simulink model "azfuz_pid"  (Simulink 7.7)
settings: Solver=ode3  StartTime=0.0  StopTime=50  FixedStep=0.1  RelTol=1e-6
PreLoadFcn:
  | load tras_char
values from neighbouring files (symbols this model uses):
  control_a = [-1,-0.975000000000000,-0.950000000000000,-0.925000000000000,-0.900000000000000,-0.875000000000000,-0.850000000000000,-0.825000000000000,-0.800000000000000,-0.775000000000000,-0.750000000000000,-0.725000000000000,-0.700000000000000,-0.675000000000000,-0.650000000000000,-0.625000000000000,-0.600000000000000,-0.575000000000000,-0.550000000000000,-0.525000000000000,-0.500000000000000,-0.4750000000000 ...(+1058 chars)    [main.m]
  force_a = [-1.11662323915155,-1.09378407342940,-1.07265330175950,-1.04325193963191,-1.01132720072323,-0.977223749190414,-0.938313974120250,-0.915271484375000,-0.878089162348878,-0.843089432210708,-0.808883264518567,-0.764209831066494,-0.722158864286485,-0.679419665506261,-0.643924317249568,-0.610622608349525,-0.566994046173359,-0.526776706201425,-0.495851299384715,-0.457681114394430,-0.413805712974957,-0.38 ...(+1125 chars)    [main.m]
  GCE = GE*(Kp-sqrt(Kp^2-4*Ki*Kd))/2/Ki    [main.m]
  GCU = Ki/GE    (= 0.001)    [main.m]
  GE = 1    [main.m]
  GU = Kd/GCE    [main.m]
  rpm_a = [-7339.45782001209,-7212.46690016528,-7085.45931302586,-6928.76328688402,-6788.57281024633,-6657.59465144230,-6511.41380896936,-6365.92031625604,-6207.93597881609,-6041.64663461541,-5911.49080716649,-5761.94058931792,-5622.99053485574,-5477.24984975964,-5308.98813100961,-5148.14194899341,-4993.59811636119,-4838.25096717246,-4657.71766075724,-4490.92806302583,-4332.56953312800,-4153.59004094051,-39 ...(+1020 chars)    [main.m]
  Ts = 0.1    [main.m]
undefined symbols (not defined in the file or in its folder): DiscIntNeverNeededParam
libraries: simulink x2, fuzblock x1
settings Model: Creator=melanholly  LastModifiedBy=melanholly
settings DataIOCC: SignalLoggingName=sigsOut
settings DebuggingCC: SaveWithParameterizedLinksMsg=none  SignalResolutionControl=TryResolveAllWithWarning  SolverPrmCheckMsg=none  MultiTaskDSMMsg=warning  MultiTaskCondExecSysMsg=none  StrictBusMsg=None
settings HardwareCC: TargetUnknown=on
settings RTWCC: IncludeERTFirstTime=on

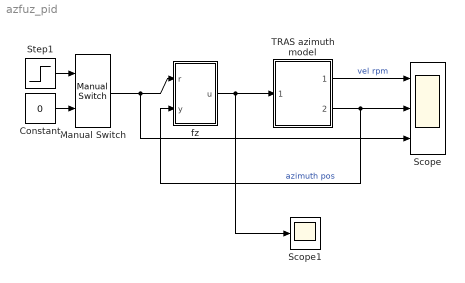
== system azfuz_pid ==
  Constant : Constant  Value=0
  Manual Switch : simulink/Signal Routing/Manual Switch  SystemSampleTime=-1  sw=1  action=0  varsize=off
  Scope : Scope  NumInputPorts=3
      settings: YMin=-5~-5~-5  YMax=5~5~5
  Scope1 : Scope
      settings: TimeRange=12  YMin=0  YMax=1.223758865248227
  Step1 : Step  After=0.3  SampleTime=0
  TRAS azimuth model : Subsystem
  fz : Subsystem
  wires:
  TRAS azimuth model/1(rpm_a) -> Scope/1  "vel rpm"
  TRAS azimuth model/2(pos_am) -> Scope/2, fz/2(y)  "azimuth pos"
  Manual Switch/1 -> Scope/3, fz/1(r)
  Step1/1 -> Manual Switch/1
  Constant/1 -> Manual Switch/2
  fz/1(u) -> TRAS azimuth model/1("ctrl_a "), Scope1/1

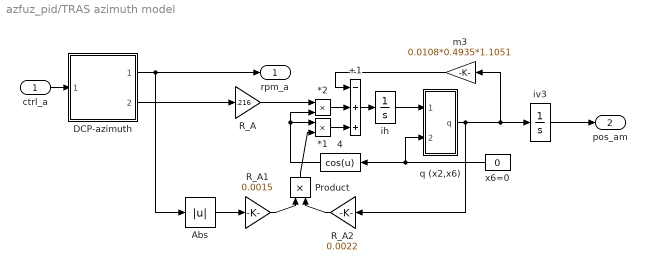
== system azfuz_pid/TRAS azimuth model ==
  "ctrl_a " : Inport
  *1 : Product  SaturateOnIntegerOverflow=on  InputSameDT=on  OutDataTypeStr=Inherit: Same as first input
  *2 : Product  SaturateOnIntegerOverflow=on  InputSameDT=on  OutDataTypeStr=Inherit: Same as first input
  +1 : Sum  Inputs=-++  SaturateOnIntegerOverflow=on  InputSameDT=on  OutDataTypeStr=Inherit: Same as first input
  4 : Fcn  Expr=cos(u)
  Abs : Abs  SaturateOnIntegerOverflow=on
  DCP-azimuth : Subsystem
  Product : Product  SaturateOnIntegerOverflow=on  InputSameDT=on  OutDataTypeStr=Inherit: Same as first input
  R_A : Gain  Gain=.216  OutDataTypeStr=Inherit: Same as input  ParamDataTypeStr=Inherit: Same as input
  R_A1 : Gain  Gain=0.0015  OutDataTypeStr=Inherit: Same as input  ParamDataTypeStr=Inherit: Same as input
  R_A2 : Gain  Gain=0.0022  OutDataTypeStr=Inherit: Same as input  ParamDataTypeStr=Inherit: Same as input
  ih : Integrator
  iv3 : Integrator
  m3 : Gain  Gain=0.0108*0.4935*1.1051  OutDataTypeStr=Inherit: Same as input  ParamDataTypeStr=Inherit: Same as input
  q (x2,x6) : Subsystem
  x6=0 : Constant  Value=0
  rpm_a : Outport
  pos_am : Outport  Port=2
  wires:
  DCP-azimuth/2(FORCE_A) -> R_A/1
  *1/1 -> +1/3
  m3/1 -> +1/1
  4/1 -> *1/1, *2/2
  *2/1 -> +1/2
  ih/1 -> q (x2,x6)/1(x2)
  q (x2,x6)/1(q) -> iv3/1, m3/1, R_A2/1
  R_A/1 -> *2/1
  +1/1 -> ih/1
  x6=0/1 -> q (x2,x6)/2(x6), 4/1
  "ctrl_a "/1 -> DCP-azimuth/1(CTR_A)
  iv3/1 -> pos_am/1
  DCP-azimuth/1(RPM_A) -> rpm_a/1, Abs/1
  Product/1 -> *1/2
  R_A2/1 -> Product/2
  R_A1/1 -> Product/1
  Abs/1 -> R_A1/1

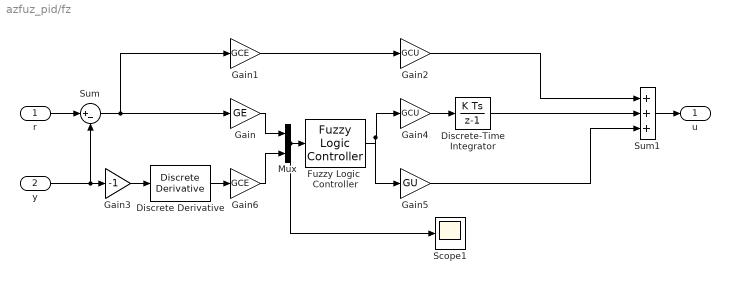
== system azfuz_pid/fz ==
  r : Inport
  y : Inport  Port=2
  Discrete Derivative : simulink/Discrete/Discrete Derivative  SystemSampleTime=-1  gainval=1.0  ICPrevScaledInput=0.0  OutMin=[]  OutMax=[]  OutDataType=fixdt(1, 16)  OutScaling=2^-10  DoSatur=off
  Discrete-Time Integrator : DiscreteIntegrator  SampleTime=Ts  ICPrevOutput=DiscIntNeverNeededParam  ICPrevScaledInput=DiscIntNeverNeededParam
  Fuzzy Logic  Controller : fuzblock/Fuzzy Logic  Controller  SystemSampleTime=-1  fis=FIS
  Gain : Gain  Gain=GE  SampleTime=Ts
  Gain1 : Gain  Gain=GCE  SampleTime=Ts
  Gain2 : Gain  Gain=GCU  SampleTime=Ts
  Gain3 : Gain  Gain=-1  SampleTime=Ts
  Gain4 : Gain  Gain=GCU  SampleTime=Ts
  Gain5 : Gain  Gain=GU  SampleTime=Ts
  Gain6 : Gain  Gain=GCE  SampleTime=Ts
  Mux : Mux  Inputs=2
  Scope1 : Scope
      settings: TimeRange=12  YMin=0  YMax=1.223758865248227  SaveName=ScopeData2
  Sum : Sum  Inputs=|+-
  Sum1 : Sum  Inputs=+++
  u : Outport
  wires:
  Gain6/1 -> Mux/2
  Gain/1 -> Mux/1
  Mux/1 -> Fuzzy Logic  Controller/1, Scope1/1
  Discrete Derivative/1 -> Gain6/1
  Gain5/1 -> Sum1/3
  Gain4/1 -> Discrete-Time Integrator/1
  Gain2/1 -> Sum1/1
  Gain1/1 -> Gain2/1
  y/1 -> Sum/2, Gain3/1
  Sum/1 -> Gain1/1, Gain/1
  Discrete-Time Integrator/1 -> Sum1/2
  Fuzzy Logic  Controller/1 -> Gain4/1, Gain5/1
  Gain3/1 -> Discrete Derivative/1
  r/1 -> Sum/1
  Sum1/1 -> u/1

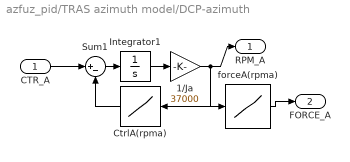
== system azfuz_pid/TRAS azimuth model/DCP-azimuth ==
  CTR_A : Inport
  1/Ja : Gain  Gain=37000  SaturateOnIntegerOverflow=on  OutDataTypeStr=Inherit: Same as input  ParamDataTypeStr=Inherit: Same as input
  CtrlA(rpma) : Lookup  InputValues=rpm_a  Table=control_a  SaturateOnIntegerOverflow=on
  Integrator1 : Integrator
  Sum1 : Sum  Inputs=|+-  SaturateOnIntegerOverflow=on  InputSameDT=on  OutDataTypeStr=Inherit: Same as first input
  forceA(rpma) : Lookup  InputValues=rpm_a  Table=force_a  SaturateOnIntegerOverflow=on
  RPM_A : Outport
  FORCE_A : Outport  Port=2
  wires:
  Sum1/1 -> Integrator1/1
  CtrlA(rpma)/1 -> Sum1/2
  Integrator1/1 -> 1/Ja/1
  1/Ja/1 -> CtrlA(rpma)/1, forceA(rpma)/1, RPM_A/1
  CTR_A/1 -> Sum1/1
  forceA(rpma)/1 -> FORCE_A/1

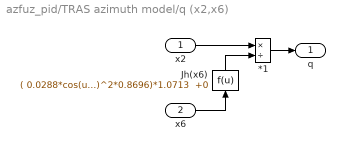
== system azfuz_pid/TRAS azimuth model/q (x2,x6) ==
  x2 : Inport
  x6 : Inport  Port=2
  " Jh(x6)" : Fcn  Expr="( 0.0288*cos(u)^2*0.8696)*1.0713  +0"
  *1 : Product  Inputs=*/  SaturateOnIntegerOverflow=on  InputSameDT=on  OutDataTypeStr=Inherit: Same as first input
  q : Outport
  wires:
  *1/1 -> q/1
  x2/1 -> *1/1
  x6/1 -> " Jh(x6)"/1
  " Jh(x6)"/1 -> *1/2
